simulink model "es2_4"  (R2022b)
settings: Solver=FixedStepDiscrete  StartTime=0.0  StopTime=30  RelTol=1e-3
values from neighbouring files (symbols this model uses):
  b = fir1(filterOrder, [low, high], 'bandpass')    [data_matrix.m]
  b_lp = fir1(filterOrder, low_cutoff, 'low')    [data_matrix.m]
libraries: vrlib x2
settings Model: Creator=simon  LastModifiedBy=franc
settings SolverCC: AlgebraicLoopSolver=TrustRegion  AutoInsertRateTranBlk=on
settings DataIOCC: LimitDataPoints=on  SaveOutput=off  SignalLogging=off  DSMLogging=off  SaveTime=off
settings OptimizationCC: ReuseModelBlockBuffer=on  LifeSpan=inf
settings DebuggingCC: AlgebraicLoopMsg=error  SingleTaskRateTransMsg=error  UnconnectedInputMsg=warning  UnconnectedOutputMsg=warning  UnconnectedLineMsg=warning  AllowSymbolicDim=off  SFUnexpectedBacktrackingDiag=warning  SFNoUnconditionalDefaultTransitionDiag=warning  SFExecutionAtInitializationDiag=none  ArithmeticOperatorsInVariantConditions=warning
settings ModelReferenceCC: EnableRefExpFcnMdlSchedulingChecks=on
settings SFSimCC: SimUseLocalCustomCode=off  CustomCodeUndefinedFunction=UseInterfaceOnly
settings RTWCC: RTWUseLocalCustomCode=off
settings CodeAppCC: StateflowObjectComments=on
settings GRTTargetCC: TargetLangStandard=C89/C90 (ANSI)

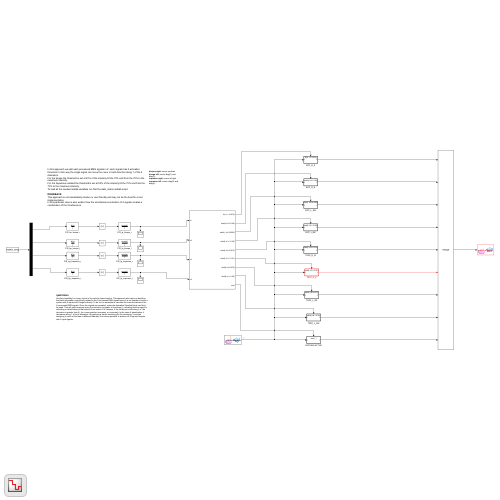
[thumbnail: Simulink's stored preview of the top-level diagram]
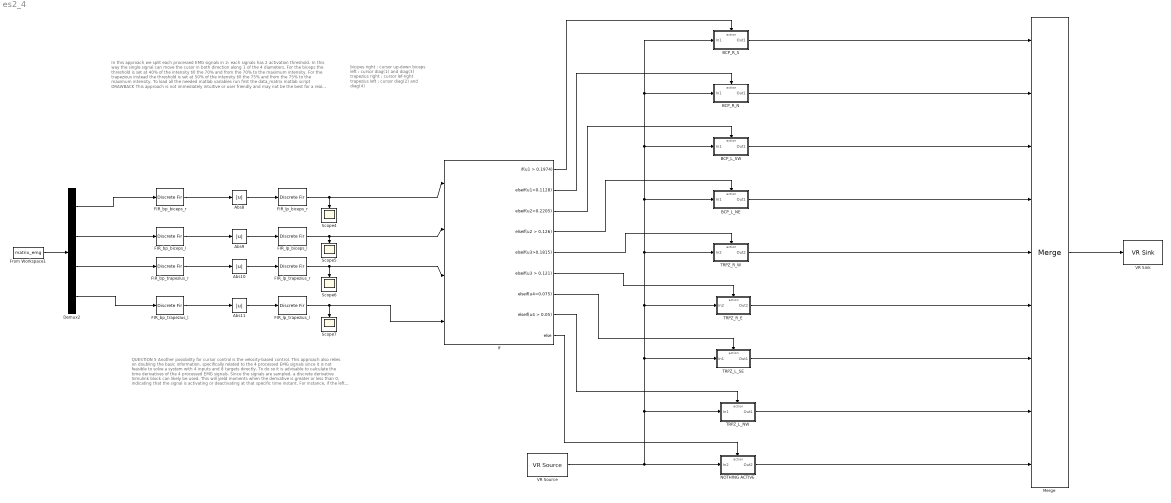
== system es2_4 ==
  note: QUESTION 5
      | Another possibility for cursor control is the velocity-based control. This approach also relies on doubling the basic information, specifically related to the 4 processed EMG signals since it is not feasible to solve a system with 4 inputs and 8 targets directly. To do so it is advisable to calculate the time derivatives of the 4 processed EMG signals. Since the signals are sampled, a discrete derivative Simulink block can likely be used. This will yield moments when the derivative is greater or less than 0, indicating that the signal is activating or deactivating at that specific time instant. For instance, if the left bicep is activating (i.e., the derivative is greater than 0), the cursor position increases, or conversely, in the case of deactivation, it decreases along 1 of the 4 diameters . By applying a similar reasoning for the remaining 3 muscles assigning to each of the them a different diameter, it becomes possible to achieve all 8 required targets with 4 input signals.
  note: bicipes right : cursor up-down
      | biceps left : cursor diag(1) and diag(3)
      | trapezius right : cursor lef-right
      | trapezius left : cursor diag(2) and diag(4)
  note: In this approach we split each processed EMG signals in 2: each signals has 2 activation threshold. In this way the single signal can move the cusor in both direction along 1 of the 4 diameters.
      | For the biceps the threshold is set at 40% of the intensity till the 70% and from the 70% to the maximum intensity.
      | For the trapezious instead the threshold is set at 50% of the intensity till the 75% and from the 75% to the maximum intensity.
      | To load all the needed matlab variables run first the data_matrix matlab script
      |
      | DRAWBACK
      | This approach is not immediately intuitive or user friendly and may not be the best for a real implementation.
      | In this particular case is also evident how the simultaneous activation of 2 signals creates a combination of the 2 behaviours.
  Abs{8..11} (4 alike) : Abs  SaturateOnIntegerOverflow=off
  BCP_L_NE : Subsystem  TreatAsAtomicUnit=on
  BCP_L_SW : Subsystem  TreatAsAtomicUnit=on
  BCP_R_N : Subsystem  TreatAsAtomicUnit=on
  BCP_R_S : Subsystem  TreatAsAtomicUnit=on
  Demux2 : Demux
  FIR_bp_biceps_l : DiscreteFir  Coefficients=b  SampleTime=1/1000
  FIR_bp_biceps_r : DiscreteFir  Coefficients=b  SampleTime=1/1000
  FIR_bp_trapezius_l : DiscreteFir  Coefficients=b  SampleTime=1/1000
  FIR_bp_trapezius_r : DiscreteFir  Coefficients=b  SampleTime=1/1000
  FIR_lp_biceps_l : DiscreteFir  Coefficients=b_lp  SampleTime=1/1000
  FIR_lp_biceps_r : DiscreteFir  Coefficients=b_lp  SampleTime=1/1000
  FIR_lp_trapezius_l : DiscreteFir  Coefficients=b_lp  SampleTime=1/1000
  FIR_lp_trapezius_r : DiscreteFir  Coefficients=b_lp  SampleTime=1/1000
  From Workspace1 : FromWorkspace  VariableName=matrix_emg  SampleTime=1/1000
  If : If  NumInputs=4  IfExpression=u1 > 0.1974  ElseIfExpressions="u1>0.1128,  u2>0.2205, u2 > 0.126, u3>0.1815, u3 > 0.121, u4>0.075, u4 > 0.05"
  Merge : Merge  Inputs=9
  NOTHING ACTIVE : Subsystem  TreatAsAtomicUnit=on
  Scope{4..7} (4 alike) : Scope
  TRPZ_L_NW : Subsystem  TreatAsAtomicUnit=on
  TRPZ_L_SE : Subsystem  TreatAsAtomicUnit=on
  TRPZ_R_E : Subsystem  TreatAsAtomicUnit=on
  TRPZ_R_W : Subsystem  TreatAsAtomicUnit=on
  VR Sink : vrlib/VR Sink  InstantiateOnLoad=on  SampleTime=1/1000  ViewEnable=on  RemoteChange=off  RemoteView=off  FieldsWritten=cursor.translation.3.1.1.double  WorldFileName=8_palline_color.wrl  AutoView=off  VideoDimensions=[]  AllowVariableSize=off  FigureProperties="{'Position', 'Name', 'Viewpoint', 'CameraBound', 'CameraDirection', 'CameraPosition', 'CameraUpVector', 'ZoomFactor', 'Antialiasing', 'Headlight', 'Lighting', 'NavPanel', 'Sound', 'StatusBar', 'Stereo3D', 'Stereo3DCameraOffset', 'Stereo3DHIT', 'ToolBar', 'Textures', 'Transparency', 'Triad', 'Wireframe', 'NavZones', 'NavMode', 'NavSpeed', 'CaptureFileFormat', 'CaptureFileName', 'Record2DCompressMethod', 'Record2DCompressQuality', 'Record2D', 'Record2DFileName', 'Record2DFPS'; [5.0000000000000000e+00   9.2200000000000045e+01   5.7600000000000000e+02   3.4999999999999994e+02], '', '_untitled_1', 'on', [0.0000000000000000e+00   0.0000000000000000e+00  -1.0000000000000000e+00], [0.0000000000000000e+00   0.0000000000000000e+00   0.0000000000000000e+00], [0.0000000000000000e+00   1.0000000000000000e+00   0.0000000000000000e+00], [1.0000000000000000e+00], 'on', 'on', 'on', 'halfbar', 'on', 'on', 'off', [1.0000000149011612e-01], [0.0000000000000000e+00], 'on', 'on', 'on', 'none', 'off', 'off', 'fly', 'normal', 'tif', '%f_anim_%n.tif', 'auto', [7.5000000000000000e+01], 'off', '%f_anim_%n.avi', 'auto'}"
  VR Source : vrlib/VR Source  InstantiateOnLoad=on  SampleTime=1/1000  ViewEnable=on  RemoteChange=off  RemoteView=off  FieldsRead=cursor.translation.1.3.1.double  WorldFileName=8_palline_color.wrl  AutoView=off  VideoDimensions=[]  AllowVariableSize=off  FigureProperties=[]
  wires:
  Abs8/1 -> FIR_lp_biceps_r/1
  FIR_bp_trapezius_r/1 -> Abs10/1
  FIR_lp_trapezius_r/1 -> Scope6/1, If/3
  FIR_lp_biceps_l/1 -> If/2, Scope5/1
  Abs11/1 -> FIR_lp_trapezius_l/1
  FIR_lp_trapezius_l/1 -> Scope7/1, If/4
  From Workspace1/1 -> Demux2/1
  Demux2/2 -> FIR_bp_biceps_l/1
  Demux2/1 -> FIR_bp_biceps_r/1
  FIR_bp_biceps_r/1 -> Abs8/1
  Demux2/3 -> FIR_bp_trapezius_r/1
  Abs9/1 -> FIR_lp_biceps_l/1
  FIR_bp_biceps_l/1 -> Abs9/1
  FIR_lp_biceps_r/1 -> If/1, Scope4/1
  Abs10/1 -> FIR_lp_trapezius_r/1
  FIR_bp_trapezius_l/1 -> Abs11/1
  Demux2/4 -> FIR_bp_trapezius_l/1
  Merge/1 -> VR Sink/1
  BCP_L_SW/1(Out1) -> Merge/3
  BCP_L_NE/1(Out1) -> Merge/4
  TRPZ_L_SE/1(Out1) -> Merge/7
  TRPZ_L_NW/1(Out1) -> Merge/8
  TRPZ_R_W/1(Out2) -> Merge/5
  TRPZ_R_E/1(Out2) -> Merge/6
  NOTHING ACTIVE/1(Out2) -> Merge/9
  VR Source/1 -> NOTHING ACTIVE/1(In2), TRPZ_L_NW/1(In1), TRPZ_L_SE/1(In1), TRPZ_R_E/1(In2), TRPZ_R_W/1(In2), BCP_L_NE/1(In1), BCP_L_SW/1(In1), BCP_R_S/1(In1), BCP_R_N/1(In1)
  BCP_R_S/1(Out1) -> Merge/1
  BCP_R_N/1(Out1) -> Merge/2
  If/1 -> BCP_R_S/Action
  If/2 -> BCP_R_N/Action
  If/3 -> BCP_L_SW/Action
  If/4 -> BCP_L_NE/Action
  If/5 -> TRPZ_R_W/Action
  If/6 -> TRPZ_R_E/Action
  If/7 -> TRPZ_L_SE/Action
  If/8 -> TRPZ_L_NW/Action
  If/9 -> NOTHING ACTIVE/Action

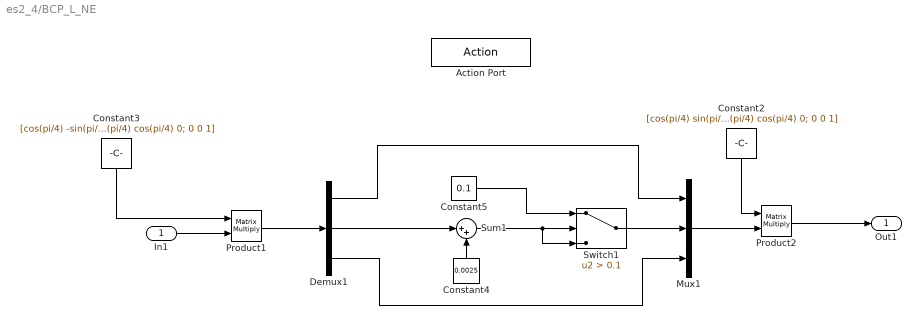
== system es2_4/BCP_L_NE ==
  In1 : Inport
  Action Port : ActionPort  ActionPortLabel=elseif( u2 > 0.126)
  Constant2 : Constant  Value=[cos(pi/4) sin(pi/4) 0; -sin(pi/4) cos(pi/4) 0; 0 0 1]  SampleTime=1/1000
  Constant3 : Constant  Value=[cos(pi/4) -sin(pi/4) 0; sin(pi/4) cos(pi/4) 0; 0 0 1]  SampleTime=1/1000
  Constant4 : Constant  Value=0.0025  SampleTime=1/1000
  Constant5 : Constant  Value=0.1  SampleTime=1/1000
  Demux1 : Demux  Outputs=3
  Mux1 : Mux  Inputs=3
  Product1 : Product  Multiplication=Matrix(*)
  Product2 : Product  Multiplication=Matrix(*)
  Sum1 : Sum  Inputs=|++  OutMin=[0]  OutMax=[0.1]
  Switch1 : Switch  Criteria=u2 > Threshold  Threshold=0.1  SaturateOnIntegerOverflow=off  InputSameDT=off
  Out1 : Outport
  wires:
  Constant2/1 -> Product2/1
  Product2/1 -> Out1/1
  Constant3/1 -> Product1/1
  In1/1 -> Product1/2
  Product1/1 -> Demux1/1
  Constant5/1 -> Switch1/1
  Switch1/1 -> Mux1/2
  Demux1/1 -> Mux1/1
  Demux1/3 -> Mux1/3
  Demux1/2 -> Sum1/1
  Constant4/1 -> Sum1/2
  Sum1/1 -> Switch1/3, Switch1/2
  Mux1/1 -> Product2/2

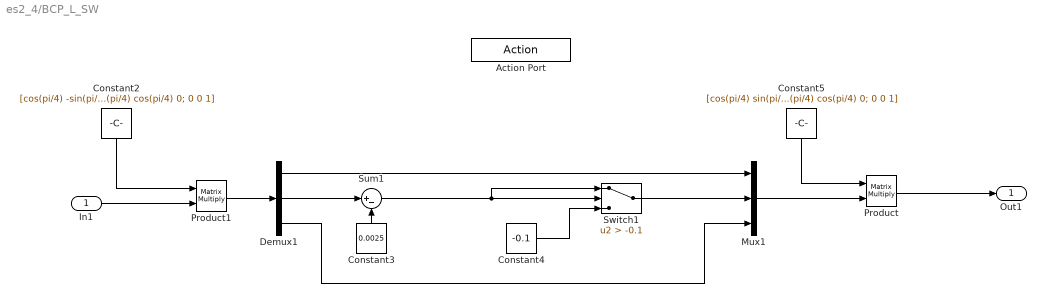
== system es2_4/BCP_L_SW ==
  In1 : Inport
  Action Port : ActionPort  ActionPortLabel="elseif(  u2>0.2205)"
  Constant2 : Constant  Value=[cos(pi/4) -sin(pi/4) 0; sin(pi/4) cos(pi/4) 0; 0 0 1]  SampleTime=1/1000
  Constant3 : Constant  Value=0.0025  SampleTime=1/1000
  Constant4 : Constant  Value=-0.1  SampleTime=1/1000
  Constant5 : Constant  Value=[cos(pi/4) sin(pi/4) 0; -sin(pi/4) cos(pi/4) 0; 0 0 1]  SampleTime=1/1000
  Demux1 : Demux  Outputs=3
  Mux1 : Mux  Inputs=3
  Product : Product  Multiplication=Matrix(*)
  Product1 : Product  Multiplication=Matrix(*)
  Sum1 : Sum  Inputs=|+-  OutMin=[-0.1]  OutMax=[0]
  Switch1 : Switch  Criteria=u2 > Threshold  Threshold=-0.1  SaturateOnIntegerOverflow=off  InputSameDT=off
  Out1 : Outport
  wires:
  Constant5/1 -> Product/1
  Mux1/1 -> Product/2
  Product/1 -> Out1/1
  Constant2/1 -> Product1/1
  In1/1 -> Product1/2
  Demux1/3 -> Mux1/3
  Sum1/1 -> Switch1/1, Switch1/2
  Constant3/1 -> Sum1/2
  Constant4/1 -> Switch1/3
  Demux1/1 -> Mux1/1
  Switch1/1 -> Mux1/2
  Demux1/2 -> Sum1/1
  Product1/1 -> Demux1/1

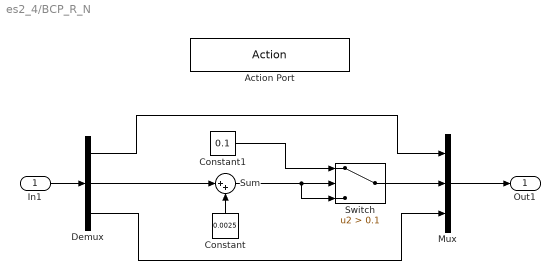
== system es2_4/BCP_R_N ==
  In1 : Inport
  Action Port : ActionPort  ActionPortLabel=elseif(u1>0.1128)
  Constant : Constant  Value=0.0025  SampleTime=1/1000
  Constant1 : Constant  Value=0.1  SampleTime=1/1000
  Demux : Demux  Outputs=3
  Mux : Mux  Inputs=3
  Sum : Sum  Inputs=|++  OutMin=[0]  OutMax=[0.1]
  Switch : Switch  Criteria=u2 > Threshold  Threshold=0.1  SaturateOnIntegerOverflow=off  InputSameDT=off
  Out1 : Outport
  wires:
  Constant/1 -> Sum/2
  Switch/1 -> Mux/2
  Mux/1 -> Out1/1
  Demux/1 -> Mux/1
  Constant1/1 -> Switch/1
  Demux/3 -> Mux/3
  Sum/1 -> Switch/3, Switch/2
  In1/1 -> Demux/1
  Demux/2 -> Sum/1

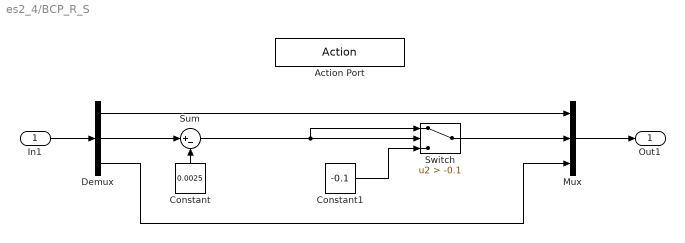
== system es2_4/BCP_R_S ==
  In1 : Inport
  Action Port : ActionPort  ActionPortLabel=if(u1 > 0.1974)
  Constant : Constant  Value=0.0025  SampleTime=1/1000
  Constant1 : Constant  Value=-0.1  SampleTime=1/1000
  Demux : Demux  Outputs=3
  Mux : Mux  Inputs=3
  Sum : Sum  Inputs=|+-  OutMin=[-0.1]  OutMax=[0]
  Switch : Switch  Criteria=u2 > Threshold  Threshold=-0.1  SaturateOnIntegerOverflow=off  InputSameDT=off
  Out1 : Outport
  wires:
  Demux/2 -> Sum/1
  Switch/1 -> Mux/2
  Demux/1 -> Mux/1
  Sum/1 -> Switch/1, Switch/2
  Demux/3 -> Mux/3
  Constant/1 -> Sum/2
  Constant1/1 -> Switch/3
  Mux/1 -> Out1/1
  In1/1 -> Demux/1

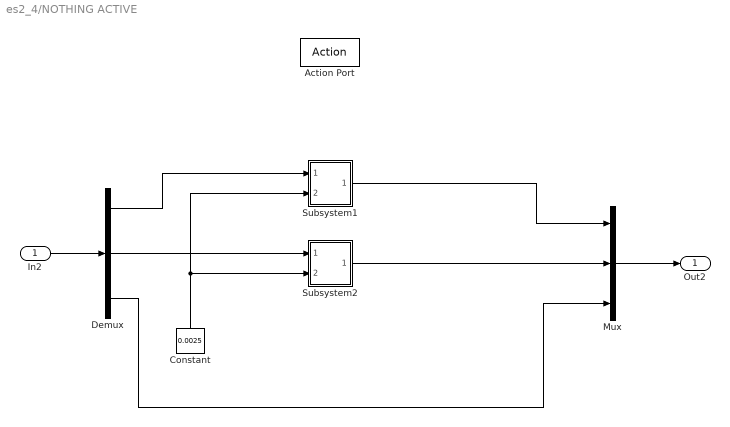
== system es2_4/NOTHING ACTIVE ==
  In2 : Inport
  Action Port : ActionPort  ActionPortLabel=else
  Constant : Constant  Value=0.0025  SampleTime=1/1000
  Demux : Demux  Outputs=3
  Mux : Mux  Inputs=3
  Subsystem1 : Subsystem
  Subsystem2 : Subsystem
  Out2 : Outport
  wires:
  Subsystem1/1(Out1) -> Mux/1
  Constant/1 -> Subsystem2/2(In2), Subsystem1/2(In2)
  Subsystem2/1(Out1) -> Mux/2
  Demux/3 -> Mux/3
  In2/1 -> Demux/1
  Mux/1 -> Out2/1
  Demux/2 -> Subsystem2/1(In1)
  Demux/1 -> Subsystem1/1(In1)

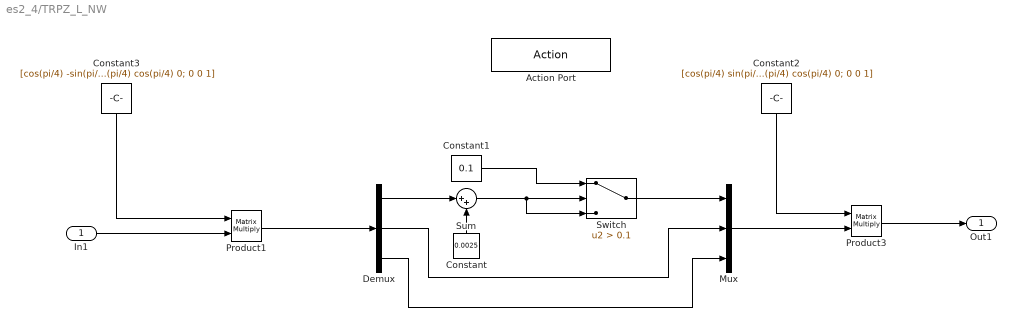
== system es2_4/TRPZ_L_NW ==
  In1 : Inport
  Action Port : ActionPort  ActionPortLabel=elseif( u4 > 0.05)
  Constant : Constant  Value=0.0025  SampleTime=1/1000
  Constant1 : Constant  Value=0.1
  Constant2 : Constant  Value=[cos(pi/4) sin(pi/4) 0; -sin(pi/4) cos(pi/4) 0; 0 0 1]  SampleTime=1/1000
  Constant3 : Constant  Value=[cos(pi/4) -sin(pi/4) 0; sin(pi/4) cos(pi/4) 0; 0 0 1]  SampleTime=1/1000
  Demux : Demux  Outputs=3
  Mux : Mux  Inputs=3
  Product1 : Product  Multiplication=Matrix(*)
  Product3 : Product  Multiplication=Matrix(*)
  Sum : Sum  Inputs=|++  OutMin=[0]  OutMax=[0.1]
  Switch : Switch  Criteria=u2 > Threshold  Threshold=0.1  SaturateOnIntegerOverflow=off  InputSameDT=off
  Out1 : Outport
  wires:
  Constant2/1 -> Product3/1
  Mux/1 -> Product3/2
  Product3/1 -> Out1/1
  Constant3/1 -> Product1/1
  In1/1 -> Product1/2
  Constant1/1 -> Switch/1
  Demux/2 -> Mux/2
  Switch/1 -> Mux/1
  Demux/1 -> Sum/1
  Demux/3 -> Mux/3
  Sum/1 -> Switch/3, Switch/2
  Constant/1 -> Sum/2
  Product1/1 -> Demux/1

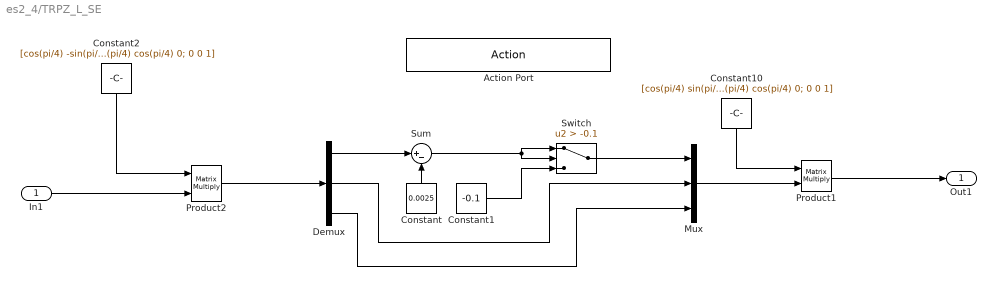
== system es2_4/TRPZ_L_SE ==
  In1 : Inport
  Action Port : ActionPort  ActionPortLabel=elseif( u4>0.075)
  Constant : Constant  Value=0.0025  SampleTime=1/1000
  Constant1 : Constant  Value=-0.1  SampleTime=1/1000
  Constant10 : Constant  Value=[cos(pi/4) sin(pi/4) 0; -sin(pi/4) cos(pi/4) 0; 0 0 1]  SampleTime=1/1000
  Constant2 : Constant  Value=[cos(pi/4) -sin(pi/4) 0; sin(pi/4) cos(pi/4) 0; 0 0 1]  SampleTime=1/1000
  Demux : Demux  Outputs=3
  Mux : Mux  Inputs=3
  Product1 : Product  Multiplication=Matrix(*)
  Product2 : Product  Multiplication=Matrix(*)
  Sum : Sum  Inputs=|+-  OutMin=[-0.1]  OutMax=[0]
  Switch : Switch  Criteria=u2 > Threshold  Threshold=-0.1  SaturateOnIntegerOverflow=off  InputSameDT=off
  Out1 : Outport
  wires:
  Constant10/1 -> Product1/1
  Mux/1 -> Product1/2
  Product1/1 -> Out1/1
  Constant2/1 -> Product2/1
  In1/1 -> Product2/2
  Sum/1 -> Switch/2, Switch/1
  Switch/1 -> Mux/1
  Demux/2 -> Mux/2
  Demux/3 -> Mux/3
  Demux/1 -> Sum/1
  Constant1/1 -> Switch/3
  Constant/1 -> Sum/2
  Product2/1 -> Demux/1

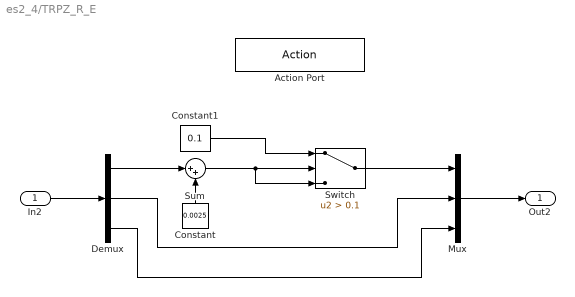
== system es2_4/TRPZ_R_E ==
  In2 : Inport
  Action Port : ActionPort  ActionPortLabel=elseif( u3 > 0.121)
  Constant : Constant  Value=0.0025  SampleTime=1/1000
  Constant1 : Constant  Value=0.1
  Demux : Demux  Outputs=3
  Mux : Mux  Inputs=3
  Sum : Sum  Inputs=|++  OutMin=[0]  OutMax=[0.1]
  Switch : Switch  Criteria=u2 > Threshold  Threshold=0.1  SaturateOnIntegerOverflow=off  InputSameDT=off
  Out2 : Outport
  wires:
  Constant1/1 -> Switch/1
  Sum/1 -> Switch/3, Switch/2
  Switch/1 -> Mux/1
  Demux/1 -> Sum/1
  Demux/3 -> Mux/3
  Constant/1 -> Sum/2
  Mux/1 -> Out2/1
  Demux/2 -> Mux/2
  In2/1 -> Demux/1

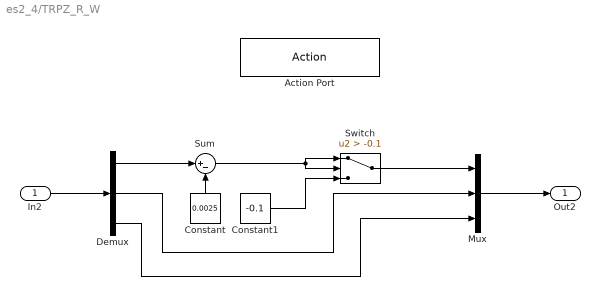
== system es2_4/TRPZ_R_W ==
  In2 : Inport
  Action Port : ActionPort  ActionPortLabel=elseif( u3>0.1815)
  Constant : Constant  Value=0.0025  SampleTime=1/1000
  Constant1 : Constant  Value=-0.1  SampleTime=1/1000
  Demux : Demux  Outputs=3
  Mux : Mux  Inputs=3
  Sum : Sum  Inputs=|+-  OutMin=[-0.1]  OutMax=[0]
  Switch : Switch  Criteria=u2 > Threshold  Threshold=-0.1  SaturateOnIntegerOverflow=off  InputSameDT=off
  Out2 : Outport
  wires:
  Sum/1 -> Switch/2, Switch/1
  Switch/1 -> Mux/1
  Demux/2 -> Mux/2
  Demux/3 -> Mux/3
  Constant/1 -> Sum/2
  Mux/1 -> Out2/1
  Demux/1 -> Sum/1
  Constant1/1 -> Switch/3
  In2/1 -> Demux/1

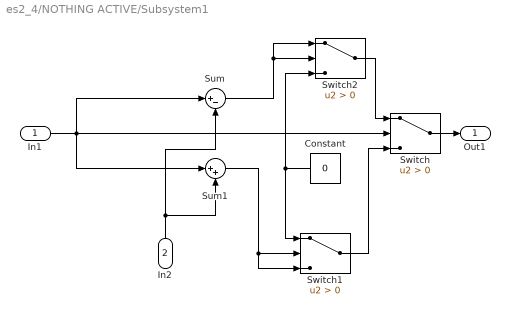
== system es2_4/NOTHING ACTIVE/Subsystem1 ==
  In1 : Inport
  In2 : Inport  Port=2
  Constant : Constant  Value=0  SampleTime=1/1000
  Sum : Sum  Inputs=|+-
  Sum1 : Sum  Inputs=|++
  Switch : Switch  Criteria=u2 > Threshold  SaturateOnIntegerOverflow=off  InputSameDT=off
  Switch1 : Switch  Criteria=u2 > Threshold  SaturateOnIntegerOverflow=off  InputSameDT=off
  Switch2 : Switch  Criteria=u2 > Threshold  SaturateOnIntegerOverflow=off  InputSameDT=off
  Out1 : Outport
  wires:
  Switch/1 -> Out1/1
  Sum1/1 -> Switch1/2, Switch1/3
  In1/1 -> Switch/2, Sum/1, Sum1/1
  In2/1 -> Sum1/2, Sum/2
  Constant/1 -> Switch2/3, Switch1/1
  Switch1/1 -> Switch/3
  Switch2/1 -> Switch/1
  Sum/1 -> Switch2/2, Switch2/1

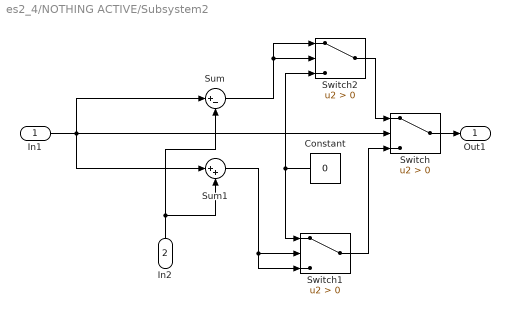
== system es2_4/NOTHING ACTIVE/Subsystem2 ==
  In1 : Inport
  In2 : Inport  Port=2
  Constant : Constant  Value=0  SampleTime=1/1000
  Sum : Sum  Inputs=|+-
  Sum1 : Sum  Inputs=|++
  Switch : Switch  Criteria=u2 > Threshold  SaturateOnIntegerOverflow=off  InputSameDT=off
  Switch1 : Switch  Criteria=u2 > Threshold  SaturateOnIntegerOverflow=off  InputSameDT=off
  Switch2 : Switch  Criteria=u2 > Threshold  SaturateOnIntegerOverflow=off  InputSameDT=off
  Out1 : Outport
  wires:
  Switch/1 -> Out1/1
  Sum1/1 -> Switch1/2, Switch1/3
  In1/1 -> Switch/2, Sum/1, Sum1/1
  In2/1 -> Sum1/2, Sum/2
  Constant/1 -> Switch2/3, Switch1/1
  Switch1/1 -> Switch/3
  Switch2/1 -> Switch/1
  Sum/1 -> Switch2/2, Switch2/1
